simulink model "PlanControlZW_cs_old"  (R2020a)
settings: Solver=ode5  StartTime=0.0  StopTime=50  FixedStep=1/1000  RelTol=1e-3
PreLoadFcn:
  | mbxruntime.callbacks.PreLoadFcn(bdroot);
PostLoadFcn:
  | mbxruntime.callbacks.PostLoadFcn(bdroot);
InitFcn:
  | mbxruntime.callbacks.InitFcn(bdroot);
StartFcn:
  | mbxruntime.callbacks.StartFcn(bdroot);
StopFcn:
  | mbxruntime.callbacks.StopFcn(bdroot);
model workspace (MAT data in the model file):
  mbox_table : object (value not decoded)
  model_closed = 0
  sim_status = 0
values from neighbouring files (symbols this model uses):
  c_factor = 43.75    [emplanner_init.m]
  cf = -175016    [emplanner_init.m]
  cr = -130634    [emplanner_init.m]
  global_path_x = [-2.22044604925e-16 0.999382255067 1.99750536558 2.99435224935 3.98991712279 4.98419835808 5.97719585569 6.96891007764 7.95934169183 8.94849144113 9.93636009523 10.9229484329 ... (501 elements, 501x1)]    [global_Path.mat]
  global_path_y = [-1.75 -1.75 -1.75 -1.75 -1.75 -1.75 -1.75 -1.75 -1.75 -1.75 -1.75 -1.75 ... (501 elements, 501x1)]    [global_Path.mat]
  KD_PID_distance = 0.0    (= 0)    [emplanner_init.m]
  KD_PID_speed = 0    [emplanner_init.m]
  KI_PID_distance = 0.0    (= 0)    [emplanner_init.m]
  KI_PID_speed = 0    [emplanner_init.m]
  KP_PID_distance = 0.5    [emplanner_init.m]
  KP_PID_speed = 1.8    [emplanner_init.m]
  la = 1.265    [emplanner_init.m]
  lb = 2.947-1.265    (= 1.682)    [emplanner_init.m]
  LQR_K1 = k(:,1)'    [emplanner_init.m]
  LQR_K2 = k(:,2)'    [emplanner_init.m]
  LQR_K3 = k(:,3)'    [emplanner_init.m]
  LQR_K4 = k(:,4)'    [emplanner_init.m]
  m = 2020    [emplanner_init.m]
  rack_displacement = [-39.14 , -37.2 , -35.29 , -33.43 , -31.6 , -29.81 , -28.06 , -26.34 , -24.66 ,      -23.01 , -21.38 , -19.79 , -18.23 , -16.69 , -15.18 , -13.7 , -12.23 , -10.8 , -9.38 , -7.98 ,     -6.61 , -5.25 , -3.91 , -2.59 , -1.29 , 0 , 1.27 , 2.54 , 3.78 , 5.02 , 6.24 , 7.46 , 8.66 ,      9.86 , 11.05 , 12.24 , 13.41 , 14.59 , 15.76 , 16.92 , 18.09 , 19.25 , 20.42 , 21.59 , 22.76 ,      23.93 , 25.11 , 26 ...(+26 chars)    [emplanner_init.m]
  right_wheel_ground = [-70 ,-67.2 , -64.4 , -61.6 , -58.8 , -56 , -53.2 , -50.4 , -47.6 , -44.8 , -42 ,      -39.2 , -36.4 , -33.6 , -30.8 , -28 , -25.2 , -22.4 , -19.6 , -16.8 , -14 , -11.2 , -8.4 , -5.6 ,      -2.8 , 0 , 2.8 , 5.6 , 8.4 , 11.2 , 14 , 16.8 , 19.6 , 22.4 , 25.2 , 28 , 30.8 , 33.6 , 36.4 ,      39.2 , 42 , 44.8 , 47.6 , 50.4 , 53.2 , 56 , 58.8 , 61.6 , 64.4 , 67.2 , 70 ]    [emplanner_init.m]
  vx_break_point = zeros(1,5000)    [emplanner_init.m]
undefined symbols (not defined in the file or in its folder): aubr, DiscIntNeverNeededParam, tablebr, vubr
libraries: PreScanSimulinkLibrary x26, simulink_extras x4, Solver_SF x1
(part 1 of 8)
CloseFcn:
  | mbxruntime.callbacks.CloseFcn(bdroot);
settings Model: Creator=PRESCAN  LastModifiedBy=Lenovo
settings DataIOCC: LimitDataPoints=on  SaveFormat=Array  SignalLoggingSaveFormat=ModelDataLogs  ReturnWorkspaceOutputs=off
settings OptimizationCC: ExpressionDepthLimit=2147483647  InitFltsAndDblsToZero=on  LifeSpan=inf
settings DebuggingCC: SaveWithParameterizedLinksMsg=none  UnderspecifiedInitializationDetection=Classic  MergeDetectMultiDrivingBlocksExec=none  SignalResolutionControl=TryResolveAllWithWarning  MultiTaskDSMMsg=warning  MultiTaskCondExecSysMsg=none  FcnCallInpInsideContextMsg=warning  StateNameClashWarn=warning  SFUnexpectedBacktrackingDiag=warning  SFNoUnconditionalDefaultTransitionDiag=warning  SFExecutionAtInitializationDiag=none  ArithmeticOperatorsInVariantConditions=warning
settings HardwareCC: ProdBitPerPointer=32  ProdBitPerSizeT=32  ProdBitPerPtrDiffT=32  ProdLargestAtomicFloat=None  ProdIntDivRoundTo=Undefined  ProdEndianess=Unspecified  ProdWordSize=32  ProdHWDeviceType=32-bit Generic
settings ModelReferenceCC: UpdateModelReferenceTargets=IfOutOfDate  PropagateSignalLabelsOutOfModel=off
settings SFSimCC: SimUseLocalCustomCode=off  SimParseCustomCode=off  CustomCodeUndefinedFunction=UseInterfaceOnly
settings SFSimCC: SimCustomHeaderCode=|
  | #include "prescan.h"
  | #include "prescan_platform.h"
settings RTWCC: RTWUseLocalCustomCode=off
settings CodeAppCC: StateflowObjectComments=on
settings GRTTargetCC: TargetFcnLib=ansi_tfl_tmw.mat  TargetLangStandard=C89/C90 (ANSI)  CombineOutputUpdateFcns=off  GRTInterface=on
settings ConfigComp: CovMetricSettings=dw  CovSaveCumulativeToWorkspaceVar=on  CovSaveSingleToWorkspaceVar=on  CovExternalEMLEnable=off

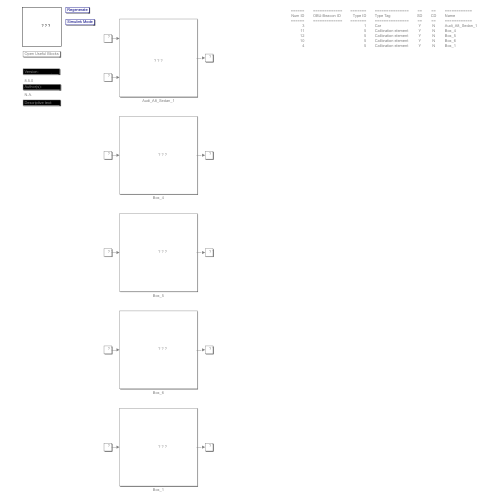
[thumbnail: Simulink's stored preview of the top-level diagram]
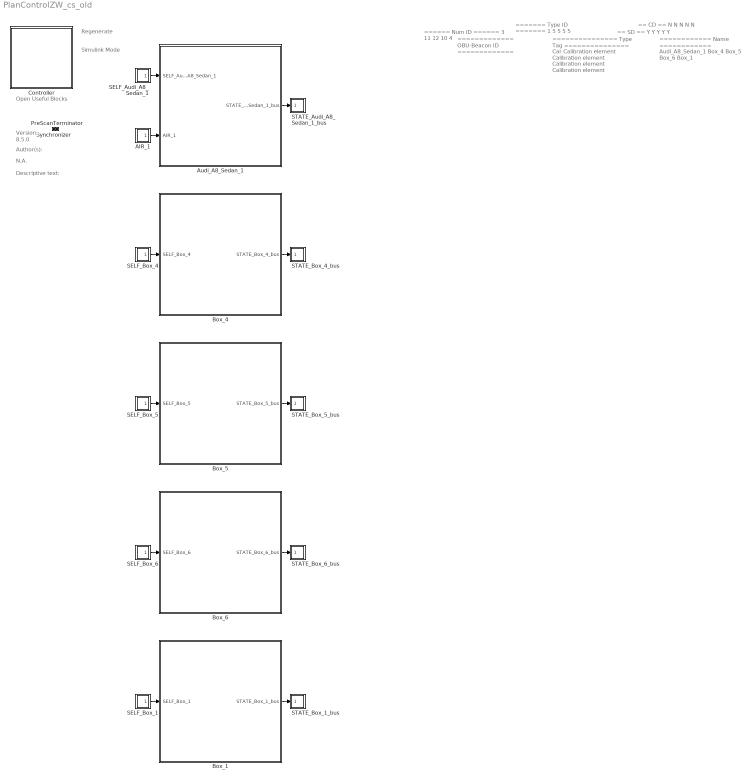
== system PlanControlZW_cs_old ==
  note: Regenerate
  note: Simulink Mode
  note: Open Useful Blocks
  note: 8.5.0
  note: Version:
  note: Author(s):
  note: N.A.
  note: Descriptive text:
  note: ======
      | Num ID
      | ======
      | 3
      | 11
      | 12
      | 10
      | 4
  note: =============
      | OBU-Beacon ID
      | =============
  note: =======
      | Type ID
      | =======
      | 1
      | 5
      | 5
      | 5
      | 5
  note: ===============
      | Type Tag
      | ===============
      | Car
      | Calibration element
      | Calibration element
      | Calibration element
      | Calibration element
  note: ==
      | SD
      | ==
      | Y
      | Y
      | Y
      | Y
      | Y
  note: ==
      | CD
      | ==
      | N
      | N
      | N
      | N
      | N
  note: ============
      | Name
      | ============
      | Audi_A8_Sedan_1
      | Box_4
      | Box_5
      | Box_6
      | Box_1
  AIR_1 : Subsystem  Tag=sensor/AIR  Priority=3  LoadFcn=load('PrescanAIRSensorData.mat');load('PrescanAIRSensorMessage.mat')  mask(PreScan Source Block: Actor Independent Receiver (AIR)){}
      mask help:
      | The Actor Information Receiver sensor provides a fast, simple and generic detection solution which is not tied up to a specific technology. The AIR detects the intersection point of the bounding box with the straight line from the sensor axis system to the middle of the bounding box.
      |
      | For more information, please click Help.
      settings: OpenFcn=open_system([gcb '/Sensor'],'mask')
      mask Help: eval('openHelp(413)')
      mask Display: image(imread('AIR.png'))
  Audi_A8_Sedan_1 : Subsystem  Tag=WorldObjectSubSystem  InitFcn=UniqueId = '15';
      mask init:
      | modelPath = GenericModelHelper.getGenericModelFilePath('ModelDepo','Vehicles\Audi_A8\Audi_A8.pgmb','d771622804618130053427da08a6d484');imagePath = GenericModelHelper.getCompilationPicture(modelPath, 'Audi_A8_HighPoly.png');
      mask Display: image(imread(imagePath));color('white');text(0, 0, ' ID=3\n')
  Box_1 : Subsystem  Tag=WorldObjectSubSystem  InitFcn=UniqueId = '690';
      mask init:
      | imagePath=which('Box.jpg');
      mask Display: image(imread(imagePath));color('white');text(0, 0, ' ID=4\n')
  Box_4 : Subsystem  Tag=WorldObjectSubSystem  InitFcn=UniqueId = '412';
      mask init:
      | imagePath=which('Box.jpg');
      mask Display: image(imread(imagePath));color('white');text(0, 0, ' ID=11\n')
  Box_5 : Subsystem  Tag=WorldObjectSubSystem  InitFcn=UniqueId = '683';
      mask init:
      | imagePath=which('Box.jpg');
      mask Display: image(imread(imagePath));color('white');text(0, 0, ' ID=12\n')
  Box_6 : Subsystem  Tag=WorldObjectSubSystem  InitFcn=UniqueId = '686';
      mask init:
      | imagePath=which('Box.jpg');
      mask Display: image(imread(imagePath));color('white');text(0, 0, ' ID=10\n')
  Controller : Subsystem  Description=0D18BAECBE05C91856EBB994EA048004049CB6BC6524C11DF47F1BB7371F592F  Priority=-1  LoadFcn=load PreScanControllerData  mask(PreScan Simulation Controller){prescanversion='8.5.0', ModelReferencing=off, TimeStep=50/1000, ControlMode=0, PreScanExecutionMode=on, ControllerCount=0, ControllerIndex=0, ControllerOptions=''}
      mask prompts: prescanversion "PreScan Version"; ModelReferencing "Use Model Referencing"; TimeStep "Upload Period [s]"; ControlMode "Control Mode"; PreScanExecutionMode "Execution Mode"; ControllerCount "Controller Count"; ControllerIndex "Controller Index"; ControllerOptions "Controller Options"
      mask help:
      | Please do not remove this block from the compilation sheet,
      | as it connects the model to the PreScan environment.
      mask init:
      | model = bdroot(gcb);
      | ExperimentFile = mbxruntime.findExperimentFile(model,true); %relative path
      | 
      | [d1, d2, d3, prescandata] = prescan_Settings();
      | ModelDepo = fullfile(prescandata,'ModelDepo'); 
      | 
      | RTmode = mbxruntime.getRTMode(model);
      | 
      | SimulationMode = get_param(bdroot,'SimulationMode');
      | if strcmp(SimulationMode, 'rapid-accelerator')
      |     SimulationMode = 'external';
      | end
      | TargetName = get_param(bdroot,'SystemTargetFile');
      settings: ModelCloseFcn=assignin('base',['model_closed_' bdroot],true);
      mask Help: eval('openHelp(812)')
      mask Display: image(imread('prescanlogo.ico'))
  PreScanTerminator : Subsystem  Tag=PreScanTerminator  Priority=999  LoadFcn=load PrescanTerminatorData  mask(PreScan Simulation Terminator){TimeStep=50/1000}
      mask prompts: TimeStep "Upload Period [s]"
      mask help:
      | Please do not remove this block from the compilation sheet as it
      | connects the model to the PreScan environment.
      mask Help: eval('openHelp(812)')
      mask Display: image(imread('prescanlogo.ico'))
  SELF_Audi_A8_Sedan_1 : Subsystem  Tag=sensor/SelfPort  Priority=3  LoadFcn=load('PreScanSelfSensorData.mat')  mask(PreScan Source Block: SELF){}
      mask help:
      | The SELF port shows (state) information of the actor itself. The outputs are position in the experiment's axis system and the GPS coordinates, and the object's absolute velocity and compass heading.
      |
      | For more information, please click Help.
      settings: OpenFcn=open_system([gcb '/Sensor'],'mask')
      mask Help: eval('openHelp(462)')
      mask Display: image(imread('GPS.png'))
  SELF_Box_1 : Subsystem  Tag=sensor/SelfPort  Priority=3  LoadFcn=load('PreScanSelfSensorData.mat')  mask(PreScan Source Block: SELF){}
      mask help:
      | The SELF port shows (state) information of the actor itself. The outputs are position in the experiment's axis system and the GPS coordinates, and the object's absolute velocity and compass heading.
      |
      | For more information, please click Help.
      settings: OpenFcn=open_system([gcb '/Sensor'],'mask')
      mask Help: eval('openHelp(462)')
      mask Display: image(imread('GPS.png'))
  SELF_Box_4 : Subsystem  Tag=sensor/SelfPort  Priority=3  LoadFcn=load('PreScanSelfSensorData.mat')  mask(PreScan Source Block: SELF){}
      mask help:
      | The SELF port shows (state) information of the actor itself. The outputs are position in the experiment's axis system and the GPS coordinates, and the object's absolute velocity and compass heading.
      |
      | For more information, please click Help.
      settings: OpenFcn=open_system([gcb '/Sensor'],'mask')
      mask Help: eval('openHelp(462)')
      mask Display: image(imread('GPS.png'))
  SELF_Box_5 : Subsystem  Tag=sensor/SelfPort  Priority=3  LoadFcn=load('PreScanSelfSensorData.mat')  mask(PreScan Source Block: SELF){}
      mask help:
      | The SELF port shows (state) information of the actor itself. The outputs are position in the experiment's axis system and the GPS coordinates, and the object's absolute velocity and compass heading.
      |
      | For more information, please click Help.
      settings: OpenFcn=open_system([gcb '/Sensor'],'mask')
      mask Help: eval('openHelp(462)')
      mask Display: image(imread('GPS.png'))
  SELF_Box_6 : Subsystem  Tag=sensor/SelfPort  Priority=3  LoadFcn=load('PreScanSelfSensorData.mat')  mask(PreScan Source Block: SELF){}
      mask help:
      | The SELF port shows (state) information of the actor itself. The outputs are position in the experiment's axis system and the GPS coordinates, and the object's absolute velocity and compass heading.
      |
      | For more information, please click Help.
      settings: OpenFcn=open_system([gcb '/Sensor'],'mask')
      mask Help: eval('openHelp(462)')
      mask Display: image(imread('GPS.png'))
  STATE_Audi_A8_Sedan_1_bus : Subsystem  Tag=actuator/StatePort  Priority=0  LoadFcn=load('PreScanStateActuatorData.mat')  mask(PreScan Sink Block: State){}
      mask help:
      | The Actor State contains a vector signal of size (9x1), containing the following signals:
      |
      | -  Position    	(x,y,z)             	[m]
      | -  Velocity    	(vx,vy,vz)         	[m/s]
      | -  Angles       	(Roll, Pitch, Yaw)	[rad]
      |
      | The Actor state is defined in the global axis system.
      | The state is superponed on the Initial position defined in the GUI.
      |
      | For more information, please click Help.
      settings: OpenFcn=open_system([gcb '/Actuator'],'mask')
      mask Help: eval('openHelp(222)')
      mask Display: image(imread('State.png'))
  STATE_Box_1_bus : Subsystem  Tag=actuator/StatePort  Priority=0  LoadFcn=load('PreScanStateActuatorData.mat')  mask(PreScan Sink Block: State){}
      mask help:
      | The Actor State contains a vector signal of size (9x1), containing the following signals:
      |
      | -  Position    	(x,y,z)             	[m]
      | -  Velocity    	(vx,vy,vz)         	[m/s]
      | -  Angles       	(Roll, Pitch, Yaw)	[rad]
      |
      | The Actor state is defined in the global axis system.
      | The state is superponed on the Initial position defined in the GUI.
      |
      | For more information, please click Help.
      settings: OpenFcn=open_system([gcb '/Actuator'],'mask')
      mask Help: eval('openHelp(222)')
      mask Display: image(imread('State.png'))
  STATE_Box_4_bus : Subsystem  Tag=actuator/StatePort  Priority=0  LoadFcn=load('PreScanStateActuatorData.mat')  mask(PreScan Sink Block: State){}
      mask help:
      | The Actor State contains a vector signal of size (9x1), containing the following signals:
      |
      | -  Position    	(x,y,z)             	[m]
      | -  Velocity    	(vx,vy,vz)         	[m/s]
      | -  Angles       	(Roll, Pitch, Yaw)	[rad]
      |
      | The Actor state is defined in the global axis system.
      | The state is superponed on the Initial position defined in the GUI.
      |
      | For more information, please click Help.
      settings: OpenFcn=open_system([gcb '/Actuator'],'mask')
      mask Help: eval('openHelp(222)')
      mask Display: image(imread('State.png'))
  STATE_Box_5_bus : Subsystem  Tag=actuator/StatePort  Priority=0  LoadFcn=load('PreScanStateActuatorData.mat')  mask(PreScan Sink Block: State){}
      mask help:
      | The Actor State contains a vector signal of size (9x1), containing the following signals:
      |
      | -  Position    	(x,y,z)             	[m]
      | -  Velocity    	(vx,vy,vz)         	[m/s]
      | -  Angles       	(Roll, Pitch, Yaw)	[rad]
      |
      | The Actor state is defined in the global axis system.
      | The state is superponed on the Initial position defined in the GUI.
      |
      | For more information, please click Help.
      settings: OpenFcn=open_system([gcb '/Actuator'],'mask')
      mask Help: eval('openHelp(222)')
      mask Display: image(imread('State.png'))
  STATE_Box_6_bus : Subsystem  Tag=actuator/StatePort  Priority=0  LoadFcn=load('PreScanStateActuatorData.mat')  mask(PreScan Sink Block: State){}
      mask help:
      | The Actor State contains a vector signal of size (9x1), containing the following signals:
      |
      | -  Position    	(x,y,z)             	[m]
      | -  Velocity    	(vx,vy,vz)         	[m/s]
      | -  Angles       	(Roll, Pitch, Yaw)	[rad]
      |
      | The Actor state is defined in the global axis system.
      | The state is superponed on the Initial position defined in the GUI.
      |
      | For more information, please click Help.
      settings: OpenFcn=open_system([gcb '/Actuator'],'mask')
      mask Help: eval('openHelp(222)')
      mask Display: image(imread('State.png'))
  Synchronizer : Subsystem  Tag=PreScanSynchronizer  Priority=1  LoadFcn=load PrescanSynchronizeData  mask(PreScan Simulation Core Block){TimeStep=50/1000}
      mask prompts: TimeStep "Timestep [s]"
      mask help:
      | Please do not remove this block from the PreScan compilation sheet,
      | as it contains essential configuration parameters for a PreScan simulation.
      settings: DeleteFcn=PreScanBlockDeleteFcn;
      mask Display: image(imread('prescanlogo.ico'))
  wires:
  Audi_A8_Sedan_1/1(STATE_Audi_A8_Sedan_1_bus) -> STATE_Audi_A8_Sedan_1_bus/1(STATE_Audi_A8_Sedan_1_bus)
  SELF_Audi_A8_Sedan_1/1(SELF_Audi_A8_Sedan_1) -> Audi_A8_Sedan_1/1(SELF_Audi_A8_Sedan_1)
  AIR_1/1(AIR_1) -> Audi_A8_Sedan_1/2(AIR_1)
  Box_4/1(STATE_Box_4_bus) -> STATE_Box_4_bus/1(STATE_Box_4_bus)
  SELF_Box_4/1(SELF_Box_4) -> Box_4/1(SELF_Box_4)
  Box_5/1(STATE_Box_5_bus) -> STATE_Box_5_bus/1(STATE_Box_5_bus)
  SELF_Box_5/1(SELF_Box_5) -> Box_5/1(SELF_Box_5)
  Box_6/1(STATE_Box_6_bus) -> STATE_Box_6_bus/1(STATE_Box_6_bus)
  SELF_Box_6/1(SELF_Box_6) -> Box_6/1(SELF_Box_6)
  Box_1/1(STATE_Box_1_bus) -> STATE_Box_1_bus/1(STATE_Box_1_bus)
  SELF_Box_1/1(SELF_Box_1) -> Box_1/1(SELF_Box_1)

== system PlanControlZW_cs_old/AIR_1 ==
  Sensor : S-Function  FunctionName=sfun_AIRSensor  Parameters=detectableObjects, sensorID, timestep  SFunctionDeploymentMode=off  EnableBusSupport=off  mask(PreScan Source Block: Actor Independent Receiver (AIR)){detectableObjects=32, sensorID=117, timestep=50/1000}
      mask prompts: detectableObjects "Max detectable objects"; sensorID "Sensor ID"; timestep "MATLAB timestep:"
      mask help:
      | The Actor Information Receiver sensor provides a fast, simple and generic detection solution which is not tied up to a specific technology. The AIR detects the intersection point of the bounding box with the straight line from the sensor axis system to the middle of the bounding box.
      |
      | For more information, please click Help.
      mask Help: eval('openHelp(413)')
      mask Display: image(imread('AIR.png'))
  AIR_1 : Outport  Tag=outport/AIR  OutDataTypeStr=Bus: PRESCAN_AIRSENSORMESSAGE  PortDimensions=32  SampleTime=50/1000
  wires:
  Sensor/1 -> AIR_1/1

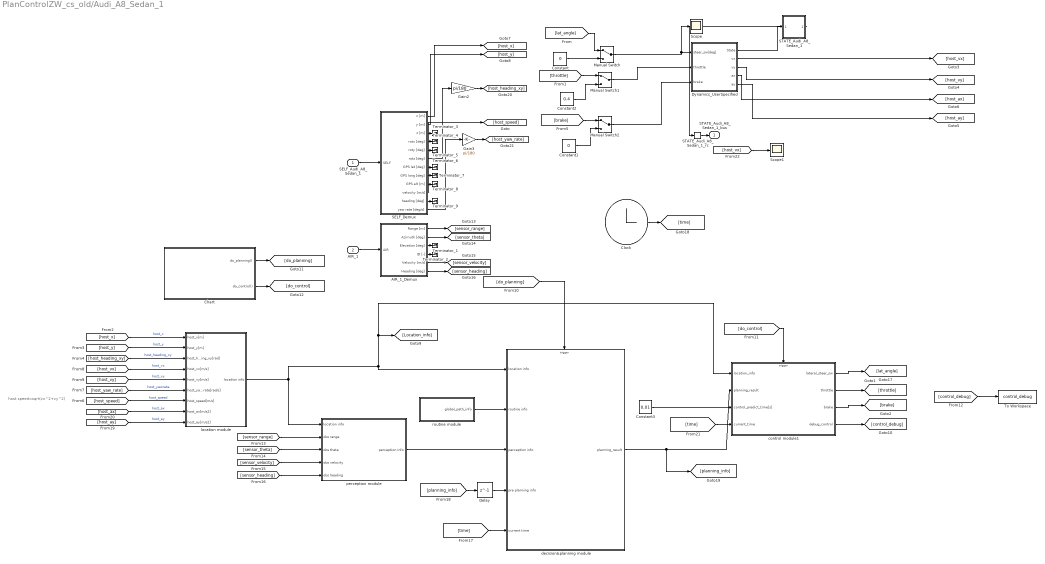
== system PlanControlZW_cs_old/Audi_A8_Sedan_1 ==
  note: host speed=sqrt(vx^2+vy^2)
  SELF_Audi_A8_Sedan_1 : Inport  Tag=inport/SelfPort  OutDataTypeStr=Bus: PRESCAN_SELFSENSORDATA  PortDimensions=1  SampleTime=50/1000  BusOutputAsStruct=on
  AIR_1 : Inport  Tag=inport/AIR  Port=2  OutDataTypeStr=Bus: PRESCAN_AIRSENSORMESSAGE  PortDimensions=32  SampleTime=50/1000  BusOutputAsStruct=on
  AIR_1_Demux : Subsystem  Tag=demux/AIR  mask(PreScan Demux Block: AIR){DetectionType=Center, detectableObjects=32}
      mask prompts: DetectionType "Detection Type"; detectableObjects "Max. detectable objects"
      mask help:
      | The Actor Information Receiver sensor provides a fast, simple and generic detection solution which is not tied up to a specific technology and can be used for scenarios in which a simple sensor is needed.
      |
      | For more information, please click Help.
      mask init:
      | switch DetectionType
      |     case 1
      |         DetectionTypeStr = 'Center';
      |     case 2
      |         DetectionTypeStr = 'BBox';
      |     case 3
      |         DetectionTypeStr = 'CoG';
      |     otherwise
      |         DetectionTypeStr = 'Unknown';
      | end
      settings: DeleteFcn=PreScanBlockDeleteFcn;
      mask Help: eval('openHelp(413)')
      mask TypeOptions DetectionType: Center | BBox | CoG
      mask Display:
      | disp(char('Det. type:         ',['{\it',DetectionTypeStr,'}']),'texmode','on')
      | port_label('output',1,'Range [m]')
      | port_label('output',2,'{\theta} [deg]','texmode','on')
      | port_label('output',3,'{\phi} [deg]','texmode','on')
      | port_label('output',4,'ID [-]','texmode','on')
      | port_label('output',5,'Velocity [m/s]','texmode','on')
      | port_label('output',6,'Heading [deg]','texmode','on')
  Chart : Stateflow chart  TreatAsAtomicUnit=on
  Clock : Clock
  Constant : Constant  Value=0
  Constant1 : Constant  Value=0
  Constant2 : Constant  Value=0.4
  Constant3 : Constant  Value=0.01
  Delay : Delay  DelayLength=1
  Dynamics_UserSpecified : Subsystem  Tag=UserSpecified_Subsys  Description=E:\002softbig\001Carsim\Prescansport\Extensions\Simulink\CarSim_VehicleDynamics.mdl  mask(User specified subsystem){update=off, sourcefilename=E:\002softbig\001Carsim\Prescansport\Extensions\Simulink\CarSim_VehicleDynamics.mdl}
      mask prompts: update "Update (default: not checked)"; sourcefilename "Source file name"
      mask help:
      | A User-specified model may be selected as Controller or Dynamics of the vehicle. PreScan will copy the contents of the User-specified model into the user-specified model block.
      |
      | If update checkbox is checked the current user-specified model block will be deleted and will be REPLACED by (new) user specified model blocks. So, the current user specified model elements will be lost.
      |
      | Warning: If a new user-specified model is selected in the GUI, the user-specified model will be replaced.
      settings: DeleteFcn=PreScanBlockDeleteFcn;
      mask Help: eval('openHelp(227)')
      mask Display: userSpecifiedDynamics_mask_display();
  Gain2 : Gain  Gain=pi/180
  Gain3 : Gain  Gain=pi/180
  Manual Switch : ManualSwitch
  Manual Switch1 : ManualSwitch
  Manual Switch2 : ManualSwitch
  SELF_Demux : Subsystem  Tag=demux/SelfPort  mask(PreScan Demux Block:){}
      mask help:
      | The SELF port shows (state) information of the actor itself. The outputs are position in the experiment's axis system and the GPS coordinates, and the object's absolute velocity and compass heading.
      |
      | For more information, please click Help.
      settings: DeleteFcn=PreScanBlockDeleteFcn;
      mask Help: eval('openHelp(462)')
      mask Display:
      | port_label('output',1,'x [m]')
      | port_label('output',2,'y [m]')
      | port_label('output',3,'z [m]','texmode','on')
      | port_label('output',4,'Rotx [deg]','texmode','on')
      | port_label('output',5,'Roty [deg]','texmode','on')
      | port_label('output',6,'Rotz [deg]','texmode','on')
      | port_label('output',7,'GPS lat [deg]','texmode','on')
      | port_label('output',8,'GPS long [deg]','texmode','on')
      | port_label('output',9,'GPS alt [m]','texmode','on')
      | port_label('output',10,'Velocity [m/s]')
      | port_label('output',11,'Heading [deg]')
      | port_label('output',12,'Yaw rate [deg/s]')
  STATE_Audi_A8_Sedan_1 : Subsystem  Tag=mux/StatePort  Priority=0  LoadFcn=load PrescanStateActuatorData  mask(PreScan Sink Block: State){x0=-1.2485, y0=4.3072, z0=0.55, Roll0=0, Pitch0=0, Yaw0=0, TimeStep=1/1000}
      mask prompts: x0 "Ini x-position VEHICLE wrt GLOBAL axis system [m]"; y0 "Ini y-position VEHICLE wrt GLOBAL axis system [m]"; z0 "Ini z-position VEHICLE wrt GLOBAL axis system [m]"; Roll0 "Ini roll-angle BODY wrt VEHICLE axis system [deg]"; Pitch0 "Ini pitch-angle BODY wrt VEHICLE axis system [deg]"; Yaw0 "Ini yaw-angle VEHICLE wrt GLOBAL axis system [deg]"; TimeStep "Auto-Assigned: Upload Period [s]"
      mask help:
      | The Actor State contains a vector signal of size (9x1), containing the following signals:
      |
      | -  Position                  (x,y,z)                                     [m]
      | -  Velocity                  (vx,vy,vz)                               [m/s]
      | -  Angles                    (Roll, Pitch, Yaw)                   [rad]
      |
      | The Actor state is defined in the global axis system.
      | The state is superponed on the Initial position defined in the GUI.
      |
      | For more information, please click Help.
      settings: DeleteFcn=PreScanBlockDeleteFcn;
      mask Help: eval('openHelp(222)')
      mask Display: image(imread('State.png'))
  STATE_Audi_A8_Sedan_1_rc : RateTransition  Tag=mux_rc/StatePort  OutPortSampleTimeOpt=Inherit
  Scope : Scope
  Scope1 : Scope
  Terminator_{1..9} (9 alike) : Terminator
  To Workspace : ToWorkspace  VariableName=control_debug  SaveFormat=Timeseries  SampleTime=-1
  control module1 : Subsystem
  decision&planning module : Subsystem
  location module : Subsystem
  perception module : Subsystem
  routine module : Subsystem
  STATE_Audi_A8_Sedan_1_bus : Outport  Tag=outport/StatePort  OutDataTypeStr=Bus: PRESCAN_STATEACTUATORDATA  PortDimensions=1  SampleTime=50/1000
  wires:
  Dynamics_UserSpecified/2(vx) -> [host_vx]
  Dynamics_UserSpecified/3(vy) -> [host_vy]
  Dynamics_UserSpecified/4(ax) -> [host_ax]
  Dynamics_UserSpecified/5(ay) -> [host_ay]
  SELF_Demux/6(rotz [deg]) -> Gain2/1
  SELF_Demux/12(yaw rate [deg/s]) -> Gain3/1
  [host_vx] -> location module/4(host_vx[m/s])  "host_vx"
  [control_debug] -> To Workspace/1
  control module1/2(throttle) -> [throttle]
  location module/1(location info) -> control module1/1(location_info), [Location_info], decision&planning module/1(location info), perception module/1(location info)
  control module1/4(debug_control) -> [control_debug]
  control module1/3(brake) -> [brake]
  [host_vy] -> location module/5(host_vy[m/s])  "host_vy"
  [host_x] -> location module/1(host_x[m])  "host_x"
  control module1/1(lateral_steer_sw) -> [lat_angle]
  [host_yaw_rate] -> location module/6(host_yawrate[rad/s])  "host_yawrate"
  [host_y] -> location module/2(host_y[m])  "host_y"
  [host_speed] -> location module/7(host_speed[m/s])  "host_speed"
  decision&planning module/1(planning_result) -> [planning_info], control module1/2(planning_result)
  [host_heading_xy] -> location module/3(host_heading_xy[rad])  "host_heading_xy"
  SELF_Demux/2(y [m]) -> [host_y]
  Gain3/1 -> [host_yaw_rate]
  SELF_Demux/1(x [m]) -> [host_x]
  Gain2/1 -> [host_heading_xy]
  SELF_Demux/10(velocity [m/s]) -> [host_speed]
  Manual Switch/1 -> Dynamics_UserSpecified/1(steer_sw[deg]), Scope/1
  Manual Switch1/1 -> Dynamics_UserSpecified/2(throttle)
  Manual Switch2/1 -> Dynamics_UserSpecified/3(brake)
  routine module/1(global_path_info) -> decision&planning module/2(routine info)
  Chart/1(do_planning()) -> [do_planning]
  Chart/2(do_control()) -> [do_control]
  [do_planning] -> decision&planning module/Trigger
  [do_control] -> control module1/Trigger
  AIR_1_Demux/1(Range [m]) -> [sensor_range]
  AIR_1_Demux/2(Azimuth [deg]) -> [sensor_theta]
  AIR_1_Demux/5(Velocity [m/s]) -> [sensor_velocity]
  AIR_1_Demux/6(Heading [deg]) -> [sensor_heading]
  [sensor_range] -> perception module/2(obs range)
  [sensor_theta] -> perception module/3(obs theta)
  [sensor_velocity] -> perception module/4(obs velocity)
  [sensor_heading] -> perception module/5(obs heading)
  perception module/1(perception info) -> decision&planning module/3(perception info)
  Clock/1 -> [time]
  [time] -> decision&planning module/5(current time)
  Delay/1 -> decision&planning module/4(pre planning info)
  [planning_info] -> Delay/1
  [host_ax] -> location module/8(host_ax[m/s2])  "host_ax"
  [host_ay] -> location module/9(host_ay[m/s2])  "host_ay"
  Constant3/1 -> control module1/3(control_predict_time[s])
  [time] -> control module1/4(current_time)
  [brake] -> Manual Switch2/1
  Constant/1 -> Manual Switch/2
  Constant1/1 -> Manual Switch2/2
  [lat_angle] -> Manual Switch/1
  [throttle] -> Manual Switch1/1
  Constant2/1 -> Manual Switch1/2
  [host_vx] -> Scope1/1
  STATE_Audi_A8_Sedan_1_rc/1 -> STATE_Audi_A8_Sedan_1_bus/1
  STATE_Audi_A8_Sedan_1/1(StateBus) -> STATE_Audi_A8_Sedan_1_rc/1
  SELF_Audi_A8_Sedan_1/1 -> SELF_Demux/1(SELF)
  AIR_1/1 -> AIR_1_Demux/1(AIR)
  Dynamics_UserSpecified/1(State) -> STATE_Audi_A8_Sedan_1/1(State)
  AIR_1_Demux/3(Elevation [deg]) -> Terminator_1/1
  AIR_1_Demux/4(ID [-]) -> Terminator_2/1
  SELF_Demux/3(z [m]) -> Terminator_3/1
  SELF_Demux/4(rotx [deg]) -> Terminator_4/1
  SELF_Demux/5(roty [deg]) -> Terminator_5/1
  SELF_Demux/7(GPS lat [deg]) -> Terminator_6/1
  SELF_Demux/8(GPS long [deg]) -> Terminator_7/1
  SELF_Demux/9(GPS alt [m]) -> Terminator_8/1
  SELF_Demux/11(heading [deg]) -> Terminator_9/1

== system PlanControlZW_cs_old/Box_1 ==
  SELF_Box_1 : Inport  Tag=inport/SelfPort  OutDataTypeStr=Bus: PRESCAN_SELFSENSORDATA  PortDimensions=1  SampleTime=50/1000  BusOutputAsStruct=on
  SELF_Demux : Subsystem  Tag=demux/SelfPort  mask(PreScan Demux Block:){}
      mask help:
      | The SELF port shows (state) information of the actor itself. The outputs are position in the experiment's axis system and the GPS coordinates, and the object's absolute velocity and compass heading.
      |
      | For more information, please click Help.
      settings: DeleteFcn=PreScanBlockDeleteFcn;
      mask Help: eval('openHelp(462)')
      mask Display:
      | port_label('output',1,'x [m]')
      | port_label('output',2,'y [m]')
      | port_label('output',3,'z [m]','texmode','on')
      | port_label('output',4,'Rotx [deg]','texmode','on')
      | port_label('output',5,'Roty [deg]','texmode','on')
      | port_label('output',6,'Rotz [deg]','texmode','on')
      | port_label('output',7,'GPS lat [deg]','texmode','on')
      | port_label('output',8,'GPS long [deg]','texmode','on')
      | port_label('output',9,'GPS alt [m]','texmode','on')
      | port_label('output',10,'Velocity [m/s]')
      | port_label('output',11,'Heading [deg]')
      | port_label('output',12,'Yaw rate [deg/s]')
  STATE_Box_1 : Subsystem  Tag=mux/StatePort  Priority=0  LoadFcn=load PrescanStateActuatorData  mask(PreScan Sink Block: State){x0=102.3107, y0=32.8881, z0=0, Roll0=0, Pitch0=0, Yaw0=270, TimeStep=50/1000}
      mask prompts: x0 "Ini x-position VEHICLE wrt GLOBAL axis system [m]"; y0 "Ini y-position VEHICLE wrt GLOBAL axis system [m]"; z0 "Ini z-position VEHICLE wrt GLOBAL axis system [m]"; Roll0 "Ini roll-angle BODY wrt VEHICLE axis system [deg]"; Pitch0 "Ini pitch-angle BODY wrt VEHICLE axis system [deg]"; Yaw0 "Ini yaw-angle VEHICLE wrt GLOBAL axis system [deg]"; TimeStep "Auto-Assigned: Upload Period [s]"
      mask help:
      | The Actor State contains a vector signal of size (9x1), containing the following signals:
      |
      | -  Position                  (x,y,z)                                     [m]
      | -  Velocity                  (vx,vy,vz)                               [m/s]
      | -  Angles                    (Roll, Pitch, Yaw)                   [rad]
      |
      | The Actor state is defined in the global axis system.
      | The state is superponed on the Initial position defined in the GUI.
      |
      | For more information, please click Help.
      settings: DeleteFcn=PreScanBlockDeleteFcn;
      mask Help: eval('openHelp(222)')
      mask Display: image(imread('State.png'))
  STATE_Box_1_rc : RateTransition  Tag=mux_rc/StatePort  OutPortSampleTimeOpt=Inherit
  Terminator_{1..12} (12 alike) : Terminator
  Trajectories : Subsystem  Tag=Trajectories  mask(PreScan Source Block: Trajectories){}
      mask help:
      | The Trajectory block contains the trajectories defined in the PreScan Experiment Editor. The output of the trajectory block is the (vehicle) State.
      |
      | For more information, please click Help.
      settings: DeleteFcn=PreScanBlockDeleteFcn;
      mask Help: eval('openHelp(312)')
      mask Display: image(imread('Trajectory.png'));
  STATE_Box_1_bus : Outport  Tag=outport/StatePort  OutDataTypeStr=Bus: PRESCAN_STATEACTUATORDATA  PortDimensions=1  SampleTime=50/1000
  wires:
  STATE_Box_1_rc/1 -> STATE_Box_1_bus/1
  STATE_Box_1/1(StateBus) -> STATE_Box_1_rc/1
  SELF_Box_1/1 -> SELF_Demux/1(SELF)
  Trajectories/1(State) -> STATE_Box_1/1(State)
  SELF_Demux/1(x [m]) -> Terminator_1/1
  SELF_Demux/2(y [m]) -> Terminator_2/1
  SELF_Demux/3(z [m]) -> Terminator_3/1
  SELF_Demux/4(rotx [deg]) -> Terminator_4/1
  SELF_Demux/5(roty [deg]) -> Terminator_5/1
  SELF_Demux/6(rotz [deg]) -> Terminator_6/1
  SELF_Demux/7(GPS lat [deg]) -> Terminator_7/1
  SELF_Demux/8(GPS long [deg]) -> Terminator_8/1
  SELF_Demux/9(GPS alt [m]) -> Terminator_9/1
  SELF_Demux/10(velocity [m/s]) -> Terminator_10/1
  SELF_Demux/11(heading [deg]) -> Terminator_11/1
  SELF_Demux/12(yaw rate [deg/s]) -> Terminator_12/1

== system PlanControlZW_cs_old/Box_4 ==
  SELF_Box_4 : Inport  Tag=inport/SelfPort  OutDataTypeStr=Bus: PRESCAN_SELFSENSORDATA  PortDimensions=1  SampleTime=50/1000  BusOutputAsStruct=on
  SELF_Demux : Subsystem  Tag=demux/SelfPort  mask(PreScan Demux Block:){}
      mask help:
      | The SELF port shows (state) information of the actor itself. The outputs are position in the experiment's axis system and the GPS coordinates, and the object's absolute velocity and compass heading.
      |
      | For more information, please click Help.
      settings: DeleteFcn=PreScanBlockDeleteFcn;
      mask Help: eval('openHelp(462)')
      mask Display:
      | port_label('output',1,'x [m]')
      | port_label('output',2,'y [m]')
      | port_label('output',3,'z [m]','texmode','on')
      | port_label('output',4,'Rotx [deg]','texmode','on')
      | port_label('output',5,'Roty [deg]','texmode','on')
      | port_label('output',6,'Rotz [deg]','texmode','on')
      | port_label('output',7,'GPS lat [deg]','texmode','on')
      | port_label('output',8,'GPS long [deg]','texmode','on')
      | port_label('output',9,'GPS alt [m]','texmode','on')
      | port_label('output',10,'Velocity [m/s]')
      | port_label('output',11,'Heading [deg]')
      | port_label('output',12,'Yaw rate [deg/s]')
  STATE_Box_4 : Subsystem  Tag=mux/StatePort  Priority=0  LoadFcn=load PrescanStateActuatorData  mask(PreScan Sink Block: State){x0=79.4828, y0=32.2235, z0=0, Roll0=0, Pitch0=0, Yaw0=270, TimeStep=50/1000}
      mask prompts: x0 "Ini x-position VEHICLE wrt GLOBAL axis system [m]"; y0 "Ini y-position VEHICLE wrt GLOBAL axis system [m]"; z0 "Ini z-position VEHICLE wrt GLOBAL axis system [m]"; Roll0 "Ini roll-angle BODY wrt VEHICLE axis system [deg]"; Pitch0 "Ini pitch-angle BODY wrt VEHICLE axis system [deg]"; Yaw0 "Ini yaw-angle VEHICLE wrt GLOBAL axis system [deg]"; TimeStep "Auto-Assigned: Upload Period [s]"
      mask help:
      | The Actor State contains a vector signal of size (9x1), containing the following signals:
      |
      | -  Position                  (x,y,z)                                     [m]
      | -  Velocity                  (vx,vy,vz)                               [m/s]
      | -  Angles                    (Roll, Pitch, Yaw)                   [rad]
      |
      | The Actor state is defined in the global axis system.
      | The state is superponed on the Initial position defined in the GUI.
      |
      | For more information, please click Help.
      settings: DeleteFcn=PreScanBlockDeleteFcn;
      mask Help: eval('openHelp(222)')
      mask Display: image(imread('State.png'))
  STATE_Box_4_rc : RateTransition  Tag=mux_rc/StatePort  OutPortSampleTimeOpt=Inherit
  Terminator_{1..12} (12 alike) : Terminator
  Trajectories : Subsystem  Tag=Trajectories  mask(PreScan Source Block: Trajectories){}
      mask help:
      | The Trajectory block contains the trajectories defined in the PreScan Experiment Editor. The output of the trajectory block is the (vehicle) State.
      |
      | For more information, please click Help.
      settings: DeleteFcn=PreScanBlockDeleteFcn;
      mask Help: eval('openHelp(312)')
      mask Display: image(imread('Trajectory.png'));
  STATE_Box_4_bus : Outport  Tag=outport/StatePort  OutDataTypeStr=Bus: PRESCAN_STATEACTUATORDATA  PortDimensions=1  SampleTime=50/1000
  wires:
  STATE_Box_4_rc/1 -> STATE_Box_4_bus/1
  STATE_Box_4/1(StateBus) -> STATE_Box_4_rc/1
  SELF_Box_4/1 -> SELF_Demux/1(SELF)
  Trajectories/1(State) -> STATE_Box_4/1(State)
  SELF_Demux/1(x [m]) -> Terminator_1/1
  SELF_Demux/2(y [m]) -> Terminator_2/1
  SELF_Demux/3(z [m]) -> Terminator_3/1
  SELF_Demux/4(rotx [deg]) -> Terminator_4/1
  SELF_Demux/5(roty [deg]) -> Terminator_5/1
  SELF_Demux/6(rotz [deg]) -> Terminator_6/1
  SELF_Demux/7(GPS lat [deg]) -> Terminator_7/1
  SELF_Demux/8(GPS long [deg]) -> Terminator_8/1
  SELF_Demux/9(GPS alt [m]) -> Terminator_9/1
  SELF_Demux/10(velocity [m/s]) -> Terminator_10/1
  SELF_Demux/11(heading [deg]) -> Terminator_11/1
  SELF_Demux/12(yaw rate [deg/s]) -> Terminator_12/1

== system PlanControlZW_cs_old/Box_5 ==
  SELF_Box_5 : Inport  Tag=inport/SelfPort  OutDataTypeStr=Bus: PRESCAN_SELFSENSORDATA  PortDimensions=1  SampleTime=50/1000  BusOutputAsStruct=on
  SELF_Demux : Subsystem  Tag=demux/SelfPort  mask(PreScan Demux Block:){}
      mask help:
      | The SELF port shows (state) information of the actor itself. The outputs are position in the experiment's axis system and the GPS coordinates, and the object's absolute velocity and compass heading.
      |
      | For more information, please click Help.
      settings: DeleteFcn=PreScanBlockDeleteFcn;
      mask Help: eval('openHelp(462)')
      mask Display:
      | port_label('output',1,'x [m]')
      | port_label('output',2,'y [m]')
      | port_label('output',3,'z [m]','texmode','on')
      | port_label('output',4,'Rotx [deg]','texmode','on')
      | port_label('output',5,'Roty [deg]','texmode','on')
      | port_label('output',6,'Rotz [deg]','texmode','on')
      | port_label('output',7,'GPS lat [deg]','texmode','on')
      | port_label('output',8,'GPS long [deg]','texmode','on')
      | port_label('output',9,'GPS alt [m]','texmode','on')
      | port_label('output',10,'Velocity [m/s]')
      | port_label('output',11,'Heading [deg]')
      | port_label('output',12,'Yaw rate [deg/s]')
  STATE_Box_5 : Subsystem  Tag=mux/StatePort  Priority=0  LoadFcn=load PrescanStateActuatorData  mask(PreScan Sink Block: State){x0=129.2769, y0=33.0819, z0=0, Roll0=0, Pitch0=0, Yaw0=270, TimeStep=50/1000}
      mask prompts: x0 "Ini x-position VEHICLE wrt GLOBAL axis system [m]"; y0 "Ini y-position VEHICLE wrt GLOBAL axis system [m]"; z0 "Ini z-position VEHICLE wrt GLOBAL axis system [m]"; Roll0 "Ini roll-angle BODY wrt VEHICLE axis system [deg]"; Pitch0 "Ini pitch-angle BODY wrt VEHICLE axis system [deg]"; Yaw0 "Ini yaw-angle VEHICLE wrt GLOBAL axis system [deg]"; TimeStep "Auto-Assigned: Upload Period [s]"
      mask help:
      | The Actor State contains a vector signal of size (9x1), containing the following signals:
      |
      | -  Position                  (x,y,z)                                     [m]
      | -  Velocity                  (vx,vy,vz)                               [m/s]
      | -  Angles                    (Roll, Pitch, Yaw)                   [rad]
      |
      | The Actor state is defined in the global axis system.
      | The state is superponed on the Initial position defined in the GUI.
      |
      | For more information, please click Help.
      settings: DeleteFcn=PreScanBlockDeleteFcn;
      mask Help: eval('openHelp(222)')
      mask Display: image(imread('State.png'))
  STATE_Box_5_rc : RateTransition  Tag=mux_rc/StatePort  OutPortSampleTimeOpt=Inherit
  Terminator_{1..12} (12 alike) : Terminator
  Trajectories : Subsystem  Tag=Trajectories  mask(PreScan Source Block: Trajectories){}
      mask help:
      | The Trajectory block contains the trajectories defined in the PreScan Experiment Editor. The output of the trajectory block is the (vehicle) State.
      |
      | For more information, please click Help.
      settings: DeleteFcn=PreScanBlockDeleteFcn;
      mask Help: eval('openHelp(312)')
      mask Display: image(imread('Trajectory.png'));
  STATE_Box_5_bus : Outport  Tag=outport/StatePort  OutDataTypeStr=Bus: PRESCAN_STATEACTUATORDATA  PortDimensions=1  SampleTime=50/1000
  wires:
  STATE_Box_5_rc/1 -> STATE_Box_5_bus/1
  STATE_Box_5/1(StateBus) -> STATE_Box_5_rc/1
  SELF_Box_5/1 -> SELF_Demux/1(SELF)
  Trajectories/1(State) -> STATE_Box_5/1(State)
  SELF_Demux/1(x [m]) -> Terminator_1/1
  SELF_Demux/2(y [m]) -> Terminator_2/1
  SELF_Demux/3(z [m]) -> Terminator_3/1
  SELF_Demux/4(rotx [deg]) -> Terminator_4/1
  SELF_Demux/5(roty [deg]) -> Terminator_5/1
  SELF_Demux/6(rotz [deg]) -> Terminator_6/1
  SELF_Demux/7(GPS lat [deg]) -> Terminator_7/1
  SELF_Demux/8(GPS long [deg]) -> Terminator_8/1
  SELF_Demux/9(GPS alt [m]) -> Terminator_9/1
  SELF_Demux/10(velocity [m/s]) -> Terminator_10/1
  SELF_Demux/11(heading [deg]) -> Terminator_11/1
  SELF_Demux/12(yaw rate [deg/s]) -> Terminator_12/1

== system PlanControlZW_cs_old/Box_6 ==
  SELF_Box_6 : Inport  Tag=inport/SelfPort  OutDataTypeStr=Bus: PRESCAN_SELFSENSORDATA  PortDimensions=1  SampleTime=50/1000  BusOutputAsStruct=on
  SELF_Demux : Subsystem  Tag=demux/SelfPort  mask(PreScan Demux Block:){}
      mask help:
      | The SELF port shows (state) information of the actor itself. The outputs are position in the experiment's axis system and the GPS coordinates, and the object's absolute velocity and compass heading.
      |
      | For more information, please click Help.
      settings: DeleteFcn=PreScanBlockDeleteFcn;
      mask Help: eval('openHelp(462)')
      mask Display:
      | port_label('output',1,'x [m]')
      | port_label('output',2,'y [m]')
      | port_label('output',3,'z [m]','texmode','on')
      | port_label('output',4,'Rotx [deg]','texmode','on')
      | port_label('output',5,'Roty [deg]','texmode','on')
      | port_label('output',6,'Rotz [deg]','texmode','on')
      | port_label('output',7,'GPS lat [deg]','texmode','on')
      | port_label('output',8,'GPS long [deg]','texmode','on')
      | port_label('output',9,'GPS alt [m]','texmode','on')
      | port_label('output',10,'Velocity [m/s]')
      | port_label('output',11,'Heading [deg]')
      | port_label('output',12,'Yaw rate [deg/s]')
  STATE_Box_6 : Subsystem  Tag=mux/StatePort  Priority=0  LoadFcn=load PrescanStateActuatorData  mask(PreScan Sink Block: State){x0=155.1591, y0=33.4731, z0=0, Roll0=0, Pitch0=0, Yaw0=270, TimeStep=50/1000}
      mask prompts: x0 "Ini x-position VEHICLE wrt GLOBAL axis system [m]"; y0 "Ini y-position VEHICLE wrt GLOBAL axis system [m]"; z0 "Ini z-position VEHICLE wrt GLOBAL axis system [m]"; Roll0 "Ini roll-angle BODY wrt VEHICLE axis system [deg]"; Pitch0 "Ini pitch-angle BODY wrt VEHICLE axis system [deg]"; Yaw0 "Ini yaw-angle VEHICLE wrt GLOBAL axis system [deg]"; TimeStep "Auto-Assigned: Upload Period [s]"
      mask help:
      | The Actor State contains a vector signal of size (9x1), containing the following signals:
      |
      | -  Position                  (x,y,z)                                     [m]
      | -  Velocity                  (vx,vy,vz)                               [m/s]
      | -  Angles                    (Roll, Pitch, Yaw)                   [rad]
      |
      | The Actor state is defined in the global axis system.
      | The state is superponed on the Initial position defined in the GUI.
      |
      | For more information, please click Help.
      settings: DeleteFcn=PreScanBlockDeleteFcn;
      mask Help: eval('openHelp(222)')
      mask Display: image(imread('State.png'))
  STATE_Box_6_rc : RateTransition  Tag=mux_rc/StatePort  OutPortSampleTimeOpt=Inherit
  Terminator_{1..12} (12 alike) : Terminator
  Trajectories : Subsystem  Tag=Trajectories  mask(PreScan Source Block: Trajectories){}
      mask help:
      | The Trajectory block contains the trajectories defined in the PreScan Experiment Editor. The output of the trajectory block is the (vehicle) State.
      |
      | For more information, please click Help.
      settings: DeleteFcn=PreScanBlockDeleteFcn;
      mask Help: eval('openHelp(312)')
      mask Display: image(imread('Trajectory.png'));
  STATE_Box_6_bus : Outport  Tag=outport/StatePort  OutDataTypeStr=Bus: PRESCAN_STATEACTUATORDATA  PortDimensions=1  SampleTime=50/1000
  wires:
  STATE_Box_6_rc/1 -> STATE_Box_6_bus/1
  STATE_Box_6/1(StateBus) -> STATE_Box_6_rc/1
  SELF_Box_6/1 -> SELF_Demux/1(SELF)
  Trajectories/1(State) -> STATE_Box_6/1(State)
  SELF_Demux/1(x [m]) -> Terminator_1/1
  SELF_Demux/2(y [m]) -> Terminator_2/1
  SELF_Demux/3(z [m]) -> Terminator_3/1
  SELF_Demux/4(rotx [deg]) -> Terminator_4/1
  SELF_Demux/5(roty [deg]) -> Terminator_5/1
  SELF_Demux/6(rotz [deg]) -> Terminator_6/1
  SELF_Demux/7(GPS lat [deg]) -> Terminator_7/1
  SELF_Demux/8(GPS long [deg]) -> Terminator_8/1
  SELF_Demux/9(GPS alt [m]) -> Terminator_9/1
  SELF_Demux/10(velocity [m/s]) -> Terminator_10/1
  SELF_Demux/11(heading [deg]) -> Terminator_11/1
  SELF_Demux/12(yaw rate [deg/s]) -> Terminator_12/1

== system PlanControlZW_cs_old/Controller ==
  Terminator : Terminator
  sfun_Controller : S-Function  FunctionName=sfun_Controller  Parameters=SParameter1, SParameter2, SParameter3, SParameter4, SParameter5, SParameter6, SParameter7, SParameter8, SParameter9, SParameter10, SampleTime  SFunctionDeploymentMode=off  EnableBusSupport=off  mask(Legacy Function){SFunctionSpec=void prescan_outputFcn(void** work1, PRESCAN_CONTROLLERDATA y1[1]), SParameter1=uint8([ExperimentFile 0]), SParameter2=uint8([ModelDepo 0]), SParameter3=uint8([ControllerOptions 0]), SParameter4=RTmode, SParameter5=PreScanExecutionMode, SParameter6=ControlMode, SParameter7=ControllerCount, SParameter8=ControllerIndex, SParameter9=uint8([SimulationMode 0]), SParameter10=uint8([TargetName 0]), SampleTime=TimeStep, ShowSpec=on}
      mask prompts: SParameter1 "P1:"; SParameter2 "P2:"; SParameter3 "P3:"; SParameter4 "P4:"; SParameter5 "P5:"; SParameter6 "P6:"; SParameter7 "P7:"; SParameter8 "P8:"; SParameter9 "P9:"; SParameter10 "P10:"; SampleTime "Sample time (-1 for inherited):"; ShowSpec "Display function specification"
      mask help:
      | This block allows you to call the legacy functions specified by the following Legacy Code Tool definition:
      | def.SFunctionName = 'sfun_Controller';
      | def.OutputFcnSpec = 'void prescan_outputFcn(void** work1, PRESCAN_CONTROLLERDATA y1[1])';
      | def.StartFcnSpec = 'void prescan_startFcn(void ** work1, uint8 p1[], uint8 p2[], uint8 p3[], double p4, double p5, double p6, double p7, double p8, uint8 p9[], uint8 p10[])';
      | def.TerminateFcnSpec = 'void prescan_terminateFcn(void** work1)';
      | def.HeaderFiles = {'prescan_controller_data.h', 'prescan_SFunLibrary.h', 'prescan_CreateLogHandler.h', 'prescan_CreateErrorHandler.h', 'prescan_modify.h', 'ModuleDLL.h'};
      | def.SourceFiles = {'prescan_MexLogHandler.c', 'prescan_SimStructErrorHandler.c', 'prescan_LogHandler.c', 'prescan_ErrorHandler.c', 'prescan_Modify.c'};
      | def.HostLibFiles = {'sensorinterfaced.lib'};
      | def.TargetLibFiles = {'sensorinterfaced.so'};
      | def.IncPaths = {'.', 'C:\projects\prescan\rt_vislibrary\vis\..\pimp\include\sensors\InterfaceRTW'};
      | def.SrcPaths = {'C:\projects\prescan\rt_vislibrary\vis\..\pimp\include\sensors\InterfaceRTW', 'C:\projects\prescan\rt_vislibrary\vis\..\pimp\include\sensors\InterfaceRTW\ccurrt'};
      | def.LibPaths = {'C:\\projects\\prescan\\vislibrary_build\lib'};
      | def.SampleTime = 'parameterized';
      mask Help: <p>This block was generated automatically by the Legacy Code Tool. For detailed help on this tool, call<a href="matlab:legacy_code('help')"> legacy_code('help')</a>.</p>
      mask Callback ShowSpec:
      | if strcmp(get_param(gcbh, 'ShowSpec'), 'on')
      |   set_param(gcbh, 'MaskDisplay', sprintf('fprintf(''%s'');', get_param(gcbh, 'SFunctionSpec')));
      | else
      |   set_param(gcbh, 'MaskDisplay', sprintf('fprintf(''%s'');', get_param(gcbh, 'FunctionName')));
      | end
      mask Display: fprintf('void prescan_outputFcn(void** work1, PRESCAN_CONTROLLERDATA y1[1])');
  wires:
  sfun_Controller/1 -> Terminator/1

== system PlanControlZW_cs_old/PreScanTerminator ==
  Terminator : Terminator
  sfun_Terminator : S-Function  FunctionName=sfun_Terminator  Parameters=SampleTime  SFunctionDeploymentMode=off  EnableBusSupport=off  mask(Legacy Function){SFunctionSpec=void prescan_terminator_outputFcn(void ** work1, PRESCAN_TERMINATORDATA y1[1]), SampleTime=TimeStep, ShowSpec=on}
      mask prompts: SampleTime "Sample time (-1 for inherited):"; ShowSpec "Display function specification"
      mask help:
      | This block allows you to call the legacy functions specified by the following Legacy Code Tool definition:
      | def.SFunctionName = 'sfun_Terminator';
      | def.OutputFcnSpec = 'void prescan_terminator_outputFcn(void ** work1, PRESCAN_TERMINATORDATA y1[1])';
      | def.StartFcnSpec = 'void prescan_terminator_startFcn(void ** work1)';
      | def.TerminateFcnSpec = 'void prescan_terminator_terminateFcn(void ** work1)';
      | def.HeaderFiles = {'prescan_terminator_data.h'};
      | def.HostLibFiles = {'sensorinterfaced.lib'};
      | def.IncPaths = {'src', 'C:\prescandev\vislibrary\vis\..\pimp\include\sensors\InterfaceRTW'};
      | def.SrcPaths = {'src'};
      | def.LibPaths = {'C:\\prescandev\\vislibrary_build\lib'};
      | def.SampleTime = 'parameterized';
      | def.Options.language = 'C';
      mask Help: <p>This block was generated automatically by the Legacy Code Tool. For detailed help on this tool, call<a href="matlab:legacy_code('help')"> legacy_code('help')</a>.</p>
      mask Callback ShowSpec:
      | if strcmp(get_param(gcbh, 'ShowSpec'), 'on')
      |   set_param(gcbh, 'MaskDisplay', sprintf('fprintf(''%s'');', get_param(gcbh, 'SFunctionSpec')));
      | else
      |   set_param(gcbh, 'MaskDisplay', sprintf('fprintf(''%s'');', get_param(gcbh, 'FunctionName')));
      | end
      mask Display: fprintf('void prescan_terminator_outputFcn(void ** work1, PRESCAN_TERMINATORDATA y1[1])');
  wires:
  sfun_Terminator/1 -> Terminator/1

== system PlanControlZW_cs_old/SELF_Audi_A8_Sedan_1 ==
  Sensor : S-Function  FunctionName=sfun_SelfSensor  Parameters=UniqueID, TimeStep  SFunctionDeploymentMode=off  EnableBusSupport=off  mask(PreScan Source Block: SELF){UniqueID=15, TimeStep=50/1000}
      mask prompts: UniqueID "Auto-Assigned: Unique ID"; TimeStep "Auto-Assigned: Upload Period [s]"
      mask help:
      | The SELF port shows (state) information of the actor itself. The outputs are position in the experiment's axis system and the GPS coordinates, and the object's absolute velocity and compass heading.
      |
      | For more information, please click Help.
      mask Help: eval('openHelp(462)')
      mask Display: image(imread('GPS.png'))
  SELF_Audi_A8_Sedan_1 : Outport  Tag=outport/SelfPort  OutDataTypeStr=Bus: PRESCAN_SELFSENSORDATA  PortDimensions=1  SampleTime=50/1000
  wires:
  Sensor/1 -> SELF_Audi_A8_Sedan_1/1

== system PlanControlZW_cs_old/SELF_Box_1 ==
  Sensor : S-Function  FunctionName=sfun_SelfSensor  Parameters=UniqueID, TimeStep  SFunctionDeploymentMode=off  EnableBusSupport=off  mask(PreScan Source Block: SELF){UniqueID=690, TimeStep=50/1000}
      mask prompts: UniqueID "Auto-Assigned: Unique ID"; TimeStep "Auto-Assigned: Upload Period [s]"
      mask help:
      | The SELF port shows (state) information of the actor itself. The outputs are position in the experiment's axis system and the GPS coordinates, and the object's absolute velocity and compass heading.
      |
      | For more information, please click Help.
      mask Help: eval('openHelp(462)')
      mask Display: image(imread('GPS.png'))
  SELF_Box_1 : Outport  Tag=outport/SelfPort  OutDataTypeStr=Bus: PRESCAN_SELFSENSORDATA  PortDimensions=1  SampleTime=50/1000
  wires:
  Sensor/1 -> SELF_Box_1/1

== system PlanControlZW_cs_old/SELF_Box_4 ==
  Sensor : S-Function  FunctionName=sfun_SelfSensor  Parameters=UniqueID, TimeStep  SFunctionDeploymentMode=off  EnableBusSupport=off  mask(PreScan Source Block: SELF){UniqueID=412, TimeStep=50/1000}
      mask prompts: UniqueID "Auto-Assigned: Unique ID"; TimeStep "Auto-Assigned: Upload Period [s]"
      mask help:
      | The SELF port shows (state) information of the actor itself. The outputs are position in the experiment's axis system and the GPS coordinates, and the object's absolute velocity and compass heading.
      |
      | For more information, please click Help.
      mask Help: eval('openHelp(462)')
      mask Display: image(imread('GPS.png'))
  SELF_Box_4 : Outport  Tag=outport/SelfPort  OutDataTypeStr=Bus: PRESCAN_SELFSENSORDATA  PortDimensions=1  SampleTime=50/1000
  wires:
  Sensor/1 -> SELF_Box_4/1
